simulink model "brusselator_sim"  (R2023a)
settings: Solver=ode1  StartTime=0.0  StopTime=600  FixedStep=0.001  RelTol=1e-3  EnableMultiTasking=on
values from neighbouring files (symbols this model uses):
  A = [0, 0, 0, 1, 0, 0; 0, 0, 0, 0, 1, 0; 0, 0, 0, 0, 0, 1; 0, 0, 0, 0, 0, 0; 0, 0, 0, 0, 0, 0; 0, 0, 0, 0, 0, 0]    [setup_lab_hover.m]
  B = [0, 0, 0 ... (first row only)    [setup_lab_hover.m]    (also in simulate_hover.m = 0.042375883612; solveSyms3.m = evalin('base', 'B'))
undefined symbols (not defined in the file or in its folder): o
libraries: dspsrcs4 x1
settings Model: ExtModeTrigDuration=10000  Creator=kille  LastModifiedBy=Jacob
settings SolverCC: AlgebraicLoopSolver=TrustRegion  PositivePriorityOrder=on  AutoInsertRateTranBlk=on
settings DataIOCC: ReturnWorkspaceOutputs=off
settings OptimizationCC: LifeSpan=inf
settings DebuggingCC: UnconnectedInputMsg=warning  UnconnectedOutputMsg=warning  UnconnectedLineMsg=warning  ArithmeticOperatorsInVariantConditions=warning
settings ModelReferenceCC: EnableRefExpFcnMdlSchedulingChecks=on
settings SFSimCC: SimUseLocalCustomCode=off  CustomCodeUndefinedFunction=UseInterfaceOnly
settings RTWCC: Description=QUARC Win64 Target  SystemTargetFile=quarc_win64.tlc  TemplateMakefile=quarc_default_tmf  RTWUseLocalCustomCode=off
settings CodeAppCC: StateflowObjectComments=on
settings STFCustomTargetCC: TargetPreCompLibLocation=C:\PROGRA~3\QUARC\lib\2016a\win64\release  UseToolchainInfoCompliant=off  SystemTargetFile=quarc_win64.tlc
settings GRTTargetCC: TargetPreCompLibLocation=C:\PROGRA~3\QUARC\lib\2016a\win64\release  ParMdlRefBuildCompliant=off  CompOptLevelCompliant=off  CombineOutputUpdateFcns=off  MatFileLogging=off  CPPClassGenCompliant=off  GRTInterface=on  UseToolchainInfoCompliant=off  ExtMode=on  ExtModeMexFile=quarc_comm
settings ConfigComp: CovMetricSettings=dswe

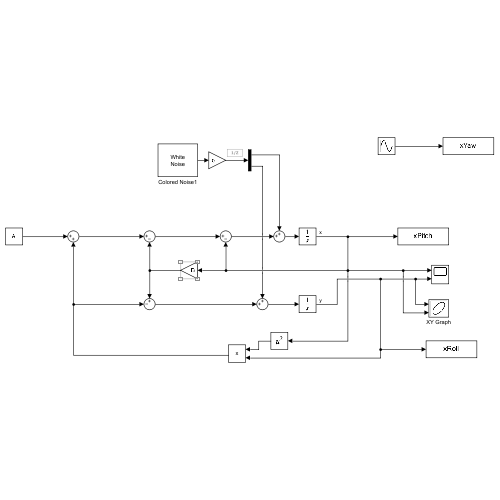
[thumbnail: Simulink's stored preview of the top-level diagram]
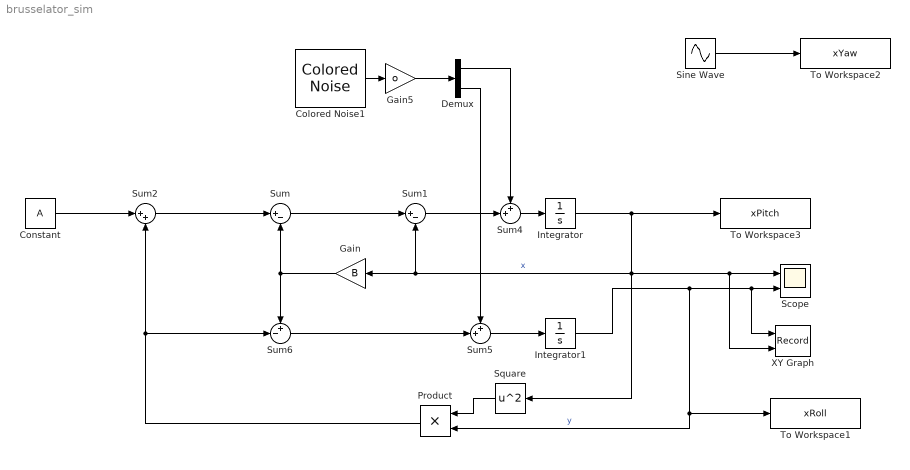
== system brusselator_sim ==
  Colored Noise1 : dspsrcs4/Colored Noise  Color=white  InverseFrequencyPower=1  BoundedOutput=off  NumChannels=2  OutputDataType=double  SamplesPerFrame=1  SampleTime=1  RandomStream=mt19937ar with seed  Seed=67  SimulateUsing=Interpreted execution
  Constant : Constant  Value=A
  Demux : Demux  Outputs=2
  Gain : Gain  Gain=B
  Gain5 : Gain  Gain=o
  Integrator : Integrator
  Integrator1 : Integrator
  Product : Product
  Scope : Scope  NumInputPorts=2
  Sine Wave : Sin  SampleTime=0
  Square : Math  Operator=square
  Sum : Sum  Inputs=|+-
  Sum1 : Sum  Inputs=|+-
  Sum2 : Sum  Inputs=|++
  Sum4 : Sum  Inputs=++|
  Sum5 : Sum  Inputs=++|
  Sum6 : Sum  Inputs=+-|
  To Workspace1 : ToWorkspace  VariableName=xRoll  SampleTime=-1
  To Workspace2 : ToWorkspace  VariableName=xYaw  SampleTime=-1
  To Workspace3 : ToWorkspace  VariableName=xPitch  SampleTime=-1
  XY Graph : Record  FileSettingsInternal="{\"entries\":[{\"content\":{\"excelSettings\":{\"content\":{},\"type\":\"Streamout.ExcelSettings\"}},\"type\":\"Streamout.FileSettingStorage\",\"uuid\":\"\"}],\"packageUris\":[\"http:\\/\\/schema.mathworks.com\\/mf0\\/streamout_blocks\\/R2020a\"],\"version\":\"1.0\"}"  Layout=[1 1]  SignalsInternal="{\"entries\":[{\"content\":{\"signals\":[{\"content\":{\"blockPath\":[],\"dimensions\":[1],\"domain\":\"\",\"lineColor\":\"#64d413\",\"plots\":[1],\"port\":1,\"sid\":[\"\"],\"signalID\":1933,\"signalName\":\"y\"},\"type\":\"RecordBlkView.Signal\",\"uuid\":\"\"},{\"content\":{\"blockPath\":[],\"dimensions\":[1],\"domain\":\"\",\"lineColor\":\"#ff13a6\",\"plots\":[1],\"port\":2,\"sid\":[\"\"],\"signalID\":1937,\"signalName\":\"x\"},\"type\":\"RecordBlkView.Signal\",\"uuid\":\"\"}]},\"type\":\"RecordBlkView.InputSignals\",\"uuid\":\"\"}],\"packageUris\":[\"http:\\/\\/schema.mathworks.com\\/mf0\\/streamout_blocks\\/R2020a\"],\"version\":\"1.0\"}"  VisualizationBindings="{\"xyplotplugin\":{\"info\":[{\"series\":[{\"bindingParametersList\":[{\"parameter\":\"X-Axis\",\"signalID\":1937,\"signalName\":\"x\"},{\"parameter\":\"Y-Axis\",\"signalID\":1933,\"signalName\":\"y\"}],\"seriesID\":18241}],\"subplotID\":1}]}}"  CompatibilityTag=XY
  wires:
  Gain5/1 -> Demux/1
  Demux/1 -> Sum4/1
  Sum4/1 -> Integrator/1
  Sum5/1 -> Integrator1/1
  Integrator1/1 -> To Workspace1/1, Product/2, XY Graph/1, Scope/2  "y"
  Colored Noise1/1 -> Gain5/1
  Integrator/1 -> To Workspace3/1, XY Graph/2, Scope/1, Square/1, Sum1/2, Gain/1  "x"
  Demux/2 -> Sum5/1
  Square/1 -> Product/1
  Product/1 -> Sum6/2, Sum2/2
  Gain/1 -> Sum6/1, Sum/2
  Constant/1 -> Sum2/1
  Sum6/1 -> Sum5/2
  Sum1/1 -> Sum4/2
  Sum/1 -> Sum1/1
  Sum2/1 -> Sum/1
  Sine Wave/1 -> To Workspace2/1
